simulink model "suggarFerm"  (R2023b)
settings: Solver=VariableStepAuto  StartTime=0.0  StopTime=10.0  RelTol=1e-3
values from neighbouring files (symbols this model uses):
  sug_current = sug_init    (= 1011.832)    [init_4_sim.m]    (also in init_sim2.m; init_sim_suggarferm.m)
  t_step = 1    [init_4_sim.m]    (also in init_sim2.m; init_sim_suggarferm.m; startingThermodynamics.m)
  temp = 296    [init_4_sim.m]    (also in init_sim.m = 298.15; init_sim2.m; init_sim_suggarferm.m)
settings Model: Creator=20181234  LastModifiedBy=20181234

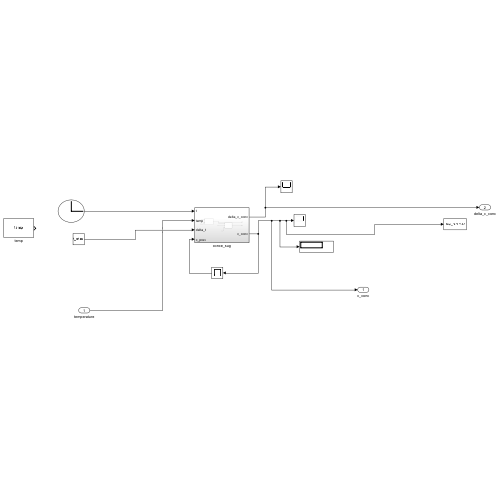
[thumbnail: Simulink's stored preview of the top-level diagram]
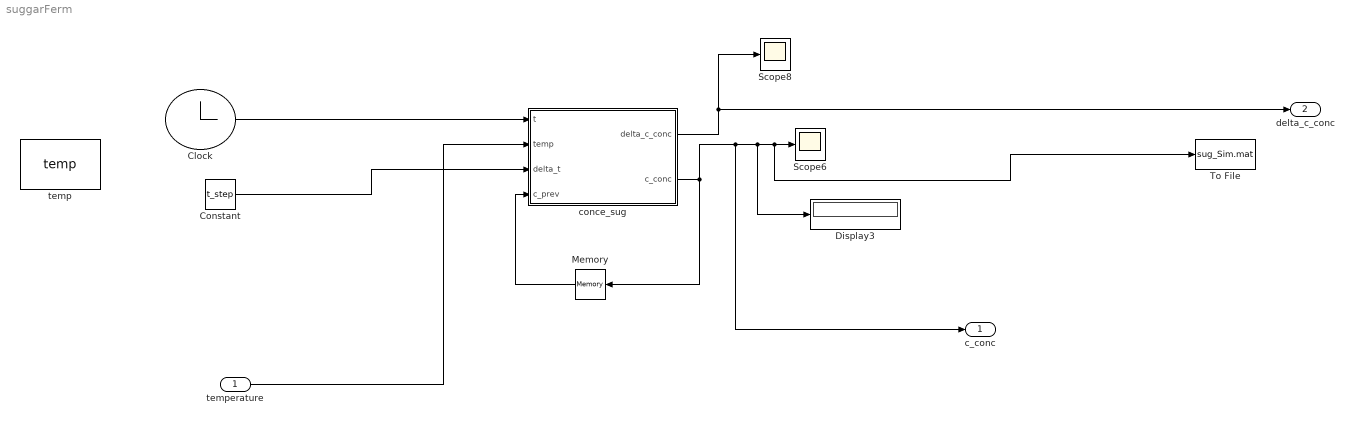
== system suggarFerm ==
  temperature : Inport
  Clock : Clock
  Constant : Constant  Value=t_step
  Display3 : Display
  Memory : Memory  InitialCondition=sug_current
  Scope6 : Scope
  Scope8 : Scope
  To File : ToFile  Filename=sug_Sim.mat  MatrixName=sug_conc
  conce_sug : Subsystem
  temp : Constant  Value=temp
  c_conc : Outport
  delta_c_conc : Outport  Port=2
  wires:
  conce_sug/1(delta_c_conc) -> Scope8/1, delta_c_conc/1
  conce_sug/2(c_conc) -> Memory/1, c_conc/1, Display3/1, To File/1, Scope6/1
  Memory/1 -> conce_sug/4(c_prev)
  Constant/1 -> conce_sug/3(delta_t)
  Clock/1 -> conce_sug/1(t)
  temperature/1 -> conce_sug/2(temp)

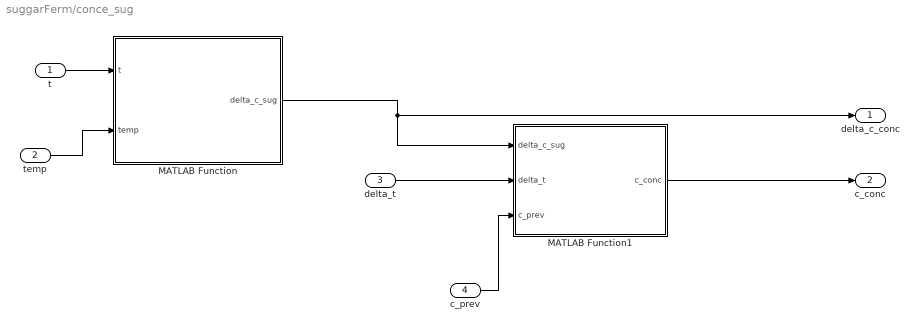
== system suggarFerm/conce_sug ==
  t : Inport
  temp : Inport  Port=2
  delta_t : Inport  Port=3
  c_prev : Inport  Port=4
  MATLAB Function : MATLAB Function  TreatAsAtomicUnit=on
  MATLAB Function1 : MATLAB Function  TreatAsAtomicUnit=on
  delta_c_conc : Outport
  c_conc : Outport  Port=2
  wires:
  MATLAB Function/1(delta_c_sug) -> delta_c_conc/1, MATLAB Function1/1(delta_c_sug)
  MATLAB Function1/1(c_conc) -> c_conc/1
  t/1 -> MATLAB Function/1(t)
  temp/1 -> MATLAB Function/2(temp)
  delta_t/1 -> MATLAB Function1/2(delta_t)
  c_prev/1 -> MATLAB Function1/3(c_prev)

== matlab function suggarFerm/conce_sug/MATLAB Function ==
  data: t input; delta_c_sug output; temp input
function delta_c_sug = dela_conc_sug(t,temp)
A = 1.24503386e-22;
E = -9.35902242e4;
m = -0.000132816;
b = -0.058764065;
R = 8.314; %j/molK

c1=A*exp(-E/(R*temp));
c2=m*temp + b;

delta_c_sug = 2*c1*t+c2;
if delta_c_sug >= 0
    delta_c_sug = 0;
end

== matlab function suggarFerm/conce_sug/MATLAB Function1 ==
  data: delta_c_sug input; c_conc output; delta_t input; c_prev input
function c_conc = c_conc_func(delta_c_sug, delta_t,c_prev)

c_conc = c_prev + delta_t*delta_c_sug;
